simulink model "pendulum_animation"  (R2022b)
settings: Solver=VariableStepAuto  StartTime=0.0  StopTime=10.0  RelTol=1e-3
undefined symbols (not defined in the file or in its folder): drawPendulum
libraries: simulink x2
settings Model: Creator=william  LastModifiedBy=william

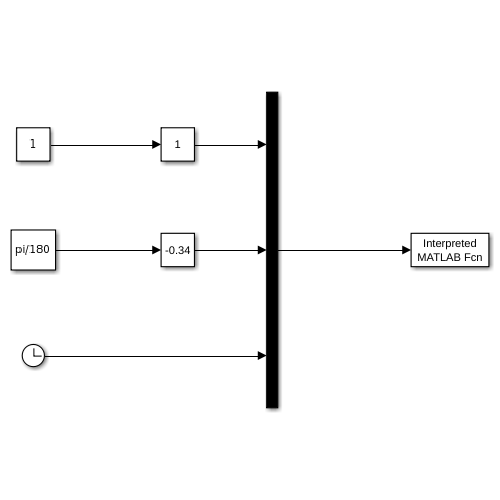
[thumbnail: Simulink's stored preview of the top-level diagram]
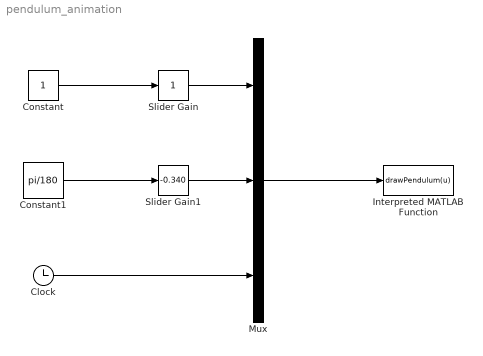
== system pendulum_animation ==
  Clock : Clock
  Constant : Constant
  Constant1 : Constant  Value=pi/180
  Interpreted MATLAB Function : MATLABFcn  MATLABFcn=drawPendulum(u)  OutputDimensions=0
  Mux : Mux  Inputs=3
  Slider Gain : simulink/Math Operations/Slider Gain  gain=1  low=-2  high=2
  Slider Gain1 : simulink/Math Operations/Slider Gain  gain=-0.340  low=-1  high=1
  wires:
  Slider Gain/1 -> Mux/1
  Slider Gain1/1 -> Mux/2
  Constant/1 -> Slider Gain/1
  Constant1/1 -> Slider Gain1/1
  Clock/1 -> Mux/3
  Mux/1 -> Interpreted MATLAB Function/1
